simulink model "exo_model_ros"  (R2020b)
settings: Solver=FixedStepAuto  StartTime=0.0  StopTime=20  FixedStep=0.002  RelTol=1e-3
undefined symbols (not defined in the file): quinientos_Hz
libraries: robotlib x12
settings Model: Creator=pablo  LastModifiedBy=pablo
settings OptimizationCC: EnhancedBackFolding=on  PassReuseOutputArgsAs=Individual arguments  ZeroExternalMemoryAtStartup=off  ZeroInternalMemoryAtStartup=off  MaxStackSize=64  OptimizeBlockOrder=speed  DifferentSizesBufferReuse=on  OptimizationCustomize=off  EfficientTunableParamExpr=on
settings DebuggingCC: ParameterTunabilityLossMsg=error
settings HardwareCC: ProdBitPerLong=64  ProdHWDeviceType=Intel->x86-64 (Linux 64)
settings SFSimCC: MATLABDynamicMemAlloc=off
settings RTWCC: Description=Embedded Coder  SystemTargetFile=ert.tlc  HardwareBoard=Robot Operating System (ROS)  TLCOptions="-aInlineSetEventsForThisBaseRateFcn=TLC_FALSE -aSuppressMultiTaskScheduler=TLC_FALSE  -aRateBasedStepFcn=0"  TemplateMakefile=ert_default_tmf  Toolchain=Catkin  TargetLang=C++
settings CodeAppCC: ForceParamTrailComments=on  IgnoreCustomStorageClasses=off  OperatorAnnotations=on  SimulinkDataObjDesc=on  SFDataObjDesc=on  InsertBlockDesc=on
settings ERTTargetCC: SupportContinuousTime=on  SupportNonInlinedSFcns=on

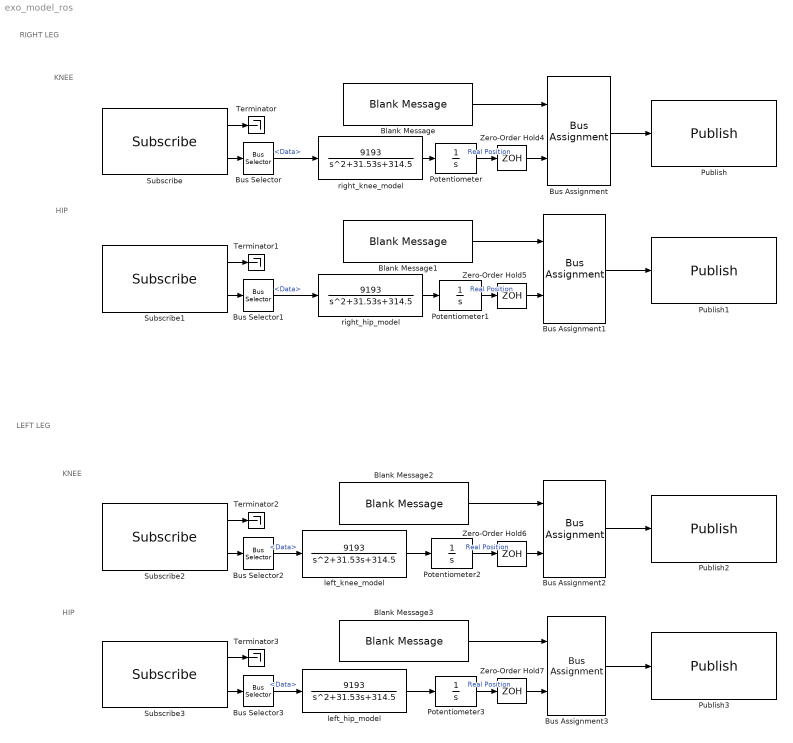
== system exo_model_ros ==
  note: HIP
  note: KNEE
  note: RIGHT LEG
  note: LEFT LEG
  note: KNEE
  note: HIP
  Blank Message{,1..3} (4 alike) : robotlib/Blank Message  messageClass=Message  entityType=std_msgs/Float64  messageType=std_msgs/Float64  SampleTime=inf  legacyBusStruct=off
  Bus Assignment{,1..3} (4 alike) : BusAssignment  AssignedSignals=Data
  Bus Selector{,1..3} (4 alike) : BusSelector  OutputSignals=Data
  Potentiometer{,1..3} (4 alike) : Integrator  InitialCondition=6
  Publish : robotlib/Publish  topicSource=Specify your own  topic=/right_knee_angle  messageType=std_msgs/Float64  legacyBusStruct=off  messageQueueLength=1
  Publish1 : robotlib/Publish  topicSource=Specify your own  topic=/right_hip_angle  messageType=std_msgs/Float64  legacyBusStruct=off  messageQueueLength=1
  Publish2 : robotlib/Publish  topicSource=Specify your own  topic=/left_knee_angle  messageType=std_msgs/Float64  legacyBusStruct=off  messageQueueLength=1
  Publish3 : robotlib/Publish  topicSource=Specify your own  topic=/left_hip_angle  messageType=std_msgs/Float64  legacyBusStruct=off  messageQueueLength=1
  Subscribe : robotlib/Subscribe  topicSource=Specify your own  topic=/right_knee_Vout  messageType=std_msgs/Float64  SampleTime=quinientos_Hz  legacyBusStruct=off  messageQueueLength=1
  Subscribe1 : robotlib/Subscribe  topicSource=Specify your own  topic=/right_hip_Vout  messageType=std_msgs/Float64  SampleTime=quinientos_Hz  legacyBusStruct=off  messageQueueLength=1
  Subscribe2 : robotlib/Subscribe  topicSource=Specify your own  topic=/left_knee_Vout  messageType=std_msgs/Float64  SampleTime=quinientos_Hz  legacyBusStruct=off  messageQueueLength=1
  Subscribe3 : robotlib/Subscribe  topicSource=Specify your own  topic=/left_hip_Vout  messageType=std_msgs/Float64  SampleTime=quinientos_Hz  legacyBusStruct=off  messageQueueLength=1
  Terminator{,1..3} (4 alike) : Terminator
  Zero-Order Hold{4..7} (4 alike) : ZeroOrderHold  SampleTime=0.002
  left_hip_model : TransferFcn  Numerator=9193  Denominator=[1 31.53 314.5]
  left_knee_model : TransferFcn  Numerator=9193  Denominator=[1 31.53 314.5]
  right_hip_model : TransferFcn  Numerator=9193  Denominator=[1 31.53 314.5]
  right_knee_model : TransferFcn  Numerator=9193  Denominator=[1 31.53 314.5]
  wires:
  Blank Message/1 -> Bus Assignment/1
  Bus Assignment/1 -> Publish/1
  Subscribe/2 -> Bus Selector/1
  right_hip_model/1 -> Potentiometer1/1
  Bus Assignment1/1 -> Publish1/1
  Blank Message1/1 -> Bus Assignment1/1
  Subscribe1/2 -> Bus Selector1/1
  Bus Selector1/1 -> right_hip_model/1  "<Data>"
  Blank Message2/1 -> Bus Assignment2/1
  left_knee_model/1 -> Potentiometer2/1
  Bus Selector3/1 -> left_hip_model/1  "<Data>"
  Subscribe3/2 -> Bus Selector3/1
  Blank Message3/1 -> Bus Assignment3/1
  Bus Assignment2/1 -> Publish2/1
  Subscribe2/2 -> Bus Selector2/1
  Bus Selector2/1 -> left_knee_model/1  "<Data>"
  left_hip_model/1 -> Potentiometer3/1
  Bus Assignment3/1 -> Publish3/1
  Subscribe/1 -> Terminator/1
  Subscribe1/1 -> Terminator1/1
  Subscribe2/1 -> Terminator2/1
  Subscribe3/1 -> Terminator3/1
  Bus Selector/1 -> right_knee_model/1  "<Data>"
  Zero-Order Hold4/1 -> Bus Assignment/2
  Zero-Order Hold5/1 -> Bus Assignment1/2
  Zero-Order Hold6/1 -> Bus Assignment2/2
  Zero-Order Hold7/1 -> Bus Assignment3/2
  right_knee_model/1 -> Potentiometer/1
  Potentiometer/1 -> Zero-Order Hold4/1  "Real Position"
  Potentiometer1/1 -> Zero-Order Hold5/1  "Real Position"
  Potentiometer2/1 -> Zero-Order Hold6/1  "Real Position"
  Potentiometer3/1 -> Zero-Order Hold7/1  "Real Position"
